simulink model "attack_decay_sim"  (R2020b)
settings: Solver=FixedStepAuto  StartTime=0.0  StopTime=simulation_time  RelTol=1e-3
InitFcn:
  | initCallback
StopFcn:
  | stopCallback
values from neighbouring files (symbols this model uses):
  band_number = 1:1:num_bands    [modelparameters.m]
  fs = 48e3    (= 48000)    [modelparameters.m]
  num_bands = 8    [modelparameters.m]
settings Model: Creator=t96f346  LastModifiedBy=conno
settings DataIOCC: ReturnWorkspaceOutputs=off

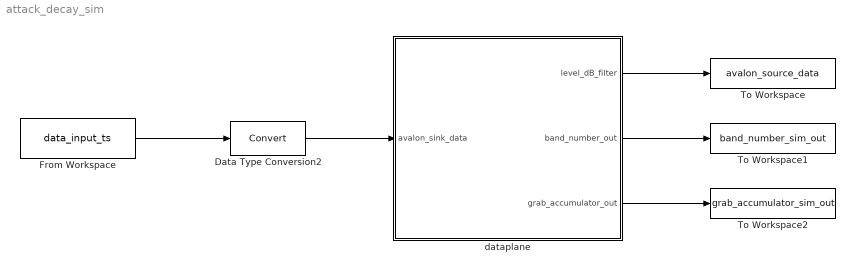
== system attack_decay_sim ==
  Data Type Conversion2 : DataTypeConversion  RndMeth=Nearest  SaturateOnIntegerOverflow=on
  From Workspace : FromWorkspace  VariableName=data_input_ts  SampleTime=1/fs
  To Workspace : ToWorkspace  VariableName=avalon_source_data  SampleTime=-1
  To Workspace1 : ToWorkspace  VariableName=band_number_sim_out  SampleTime=-1
  To Workspace2 : ToWorkspace  VariableName=grab_accumulator_sim_out  SampleTime=-1
  dataplane : Subsystem  TreatAsAtomicUnit=on
  wires:
  From Workspace/1 -> Data Type Conversion2/1
  Data Type Conversion2/1 -> dataplane/1(avalon_sink_data)
  dataplane/1(level_dB_filter) -> To Workspace/1
  dataplane/2(band_number_out) -> To Workspace1/1
  dataplane/3(grab_accumulator_out) -> To Workspace2/1

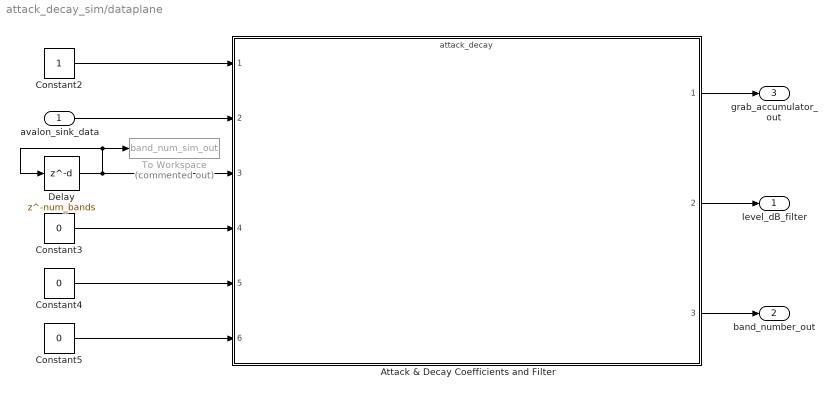
== system attack_decay_sim/dataplane ==
  avalon_sink_data : Inport  OutDataTypeStr=input_type
  Attack & Decay Coefficients and Filter : ModelReference  ModelNameDialog=attack_decay.slx  SimulationMode=Normal  ModelReferenceVersion=2.90
  Constant2 : Constant  OutDataTypeStr=boolean  SampleTime=-1
  Constant3 : Constant  Value=0  OutDataTypeStr=Inherit: Inherit via back propagation  SampleTime=-1
  Constant4 : Constant  Value=0  OutDataTypeStr=Inherit: Inherit via back propagation  SampleTime=-1
  Constant5 : Constant  Value=0  OutDataTypeStr=Inherit: Inherit via back propagation  SampleTime=-1
  Delay : Delay  DelayLength=num_bands  InitialCondition=band_number
  To Workspace : ToWorkspace  Commented=on  VariableName=band_num_sim_out  SampleTime=-1
  level_dB_filter : Outport  OutDataTypeStr=input_type  VectorParamsAs1DForOutWhenUnconnected=off
  band_number_out : Outport  Port=2
  grab_accumulator_out : Outport  Port=3
  wires:
  Constant2/1 -> Attack & Decay Coefficients and Filter/1
  Constant3/1 -> Attack & Decay Coefficients and Filter/4
  Constant5/1 -> Attack & Decay Coefficients and Filter/6
  Constant4/1 -> Attack & Decay Coefficients and Filter/5
  Attack & Decay Coefficients and Filter/1 -> grab_accumulator_out/1
  Attack & Decay Coefficients and Filter/3 -> band_number_out/1
  Delay/1 -> To Workspace/1, Delay/1, Attack & Decay Coefficients and Filter/3
  avalon_sink_data/1 -> Attack & Decay Coefficients and Filter/2
  Attack & Decay Coefficients and Filter/2 -> level_dB_filter/1
